simulink model "gnc"  (R2025b)
settings: Solver=ode2  StartTime=0.0  StopTime=inf  FixedStep=1/100  RelTol=1e-3
PreLoadFcn:
  | gnc_PreLoadFcn
undefined symbols (not defined in the file or in its folder): DiscIntNeverNeededParam, dspblkCoreblockFVToolHelper, gcbh
libraries: simulink_extras x7, simulink x5, eeGeneralControl x5
(part 1 of 4)
settings Model: Creator=ac112430  LastModifiedBy=ac124458
settings SolverCC: AlgebraicLoopSolver=TrustRegion
settings DataIOCC: ReturnWorkspaceOutputs=off
settings OptimizationCC: DefaultParameterBehavior=Inlined  DefaultUnderspecifiedDataType=single  PassReuseOutputArgsAs=Individual arguments  DifferentSizesBufferReuse=on  EfficientTunableParamExpr=on
settings DebuggingCC: ParameterPrecisionLossMsg=none  ParameterTunabilityLossMsg=error  UnconnectedInputMsg=warning  UnconnectedOutputMsg=warning  UnconnectedLineMsg=warning  BusObjectLabelMismatch=none  ArithmeticOperatorsInVariantConditions=warning
settings HardwareCC: ProdBitPerPointer=32.0  ProdBitPerSizeT=32.0  ProdBitPerPtrDiffT=32.0  ProdLargestAtomicInteger=Long  ProdLargestAtomicFloat=Double  ProdIntDivRoundTo=Undefined  ProdWordSize=32.0  ProdLongLongMode=on  ProdHWDeviceType=ARM Compatible->ARM Cortex
settings ModelReferenceCC: EnableRefExpFcnMdlSchedulingChecks=on  ModelReferenceNumInstancesAllowed=Single  PropagateSignalLabelsOutOfModel=off
settings SFSimCC: SimUseLocalCustomCode=off  MATLABDynamicMemAlloc=off  CustomCodeUndefinedFunction=UseInterfaceOnly
settings RTWCC: SystemTargetFile=ert.tlc  GenCodeOnly=on  TemplateMakefile=ert_default_tmf  RTWUseLocalCustomCode=off  IncludeHyperlinkInReport=on  GPUComputeCapability=3.5  Description=Embedded Coder
settings CodeAppCC: IgnoreCustomStorageClasses=off  MaxIdLength=2048.0  StateflowObjectComments=on
settings ERTTargetCC: ERTCustomFileTemplate=example_file_process.tlc  ConvertIfToSwitch=off  SuppressUnreachableDefaultCases=off  DynamicArrayContainerType=coder::array  TargetLangStandard=C99 (ISO)  GenerateSampleERTMain=on  SupportComplex=off  SupportVariableSizeSignals=on

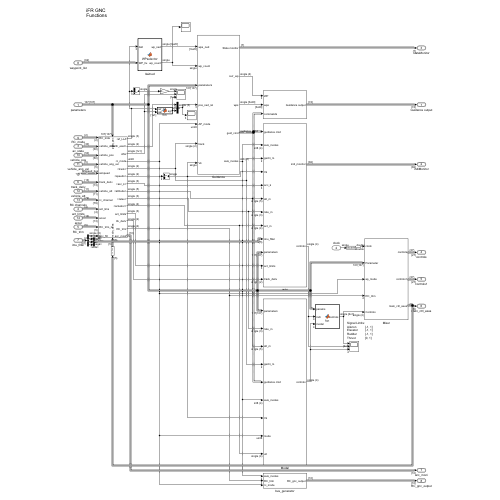
[thumbnail: Simulink's stored preview of the top-level diagram]
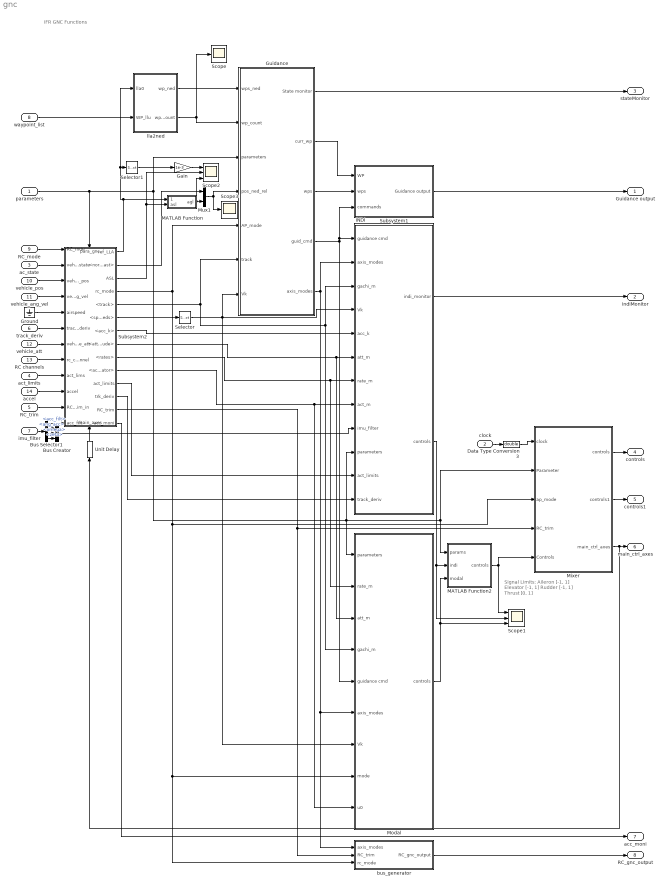
== system gnc ==
  note: iFR GNC Functions
  note: Signal Limits:
      | Aileron		[-1, 1]
      | Elevator		[-1, 1]
      | Rudder		[-1, 1]
      | Thrust		[0, 1]
  parameters : Inport  OutDataTypeStr=Bus: gnc_parameterBus
  clock : Inport  Port=2  OutDataTypeStr=single
  ac_state : Inport  Port=3  OutDataTypeStr=Bus: vehicle_state_bus  PortDimensions=1  SampleTime=[0.01,0]
  act_limits : Inport  Port=4  OutDataTypeStr=Bus: actuator_limits_bus
  RC_trim : Inport  Port=5  OutDataTypeStr=Bus: rc_trim_bus
  track_deriv : Inport  Port=6  OutDataTypeStr=Bus: track_deriv_monitor_bus
  imu_filter : Inport  Port=7  OutDataTypeStr=Bus: ifr_imu_filtered_bus
  waypoint_list : Inport  Port=8  OutDataTypeStr=Bus: waypoint_list_bus
  RC_mode : Inport  Port=9  OutDataTypeStr=Bus: rc_mode_bus
  vehicle_pos : Inport  Port=10  OutDataTypeStr=Bus: vehicle_local_position_bus
  vehicle_ang_vel : Inport  Port=11  OutDataTypeStr=Bus: vehicle_angular_velocity_bus
  vehicle_att : Inport  Port=12  OutDataTypeStr=Bus: vehicle_attitude_bus
  RC channels : Inport  Port=13  OutDataTypeStr=Bus: rc_channels_bus
  accel : Inport  Port=14  OutDataTypeStr=Bus: sensor_accel_bus
  Bus Creator : BusCreator  Inputs=3
  Bus Selector1 : BusSelector  OutputSignals=acc_filt,ang_acc,omega,zeta
  Data Type Conversion3 : DataTypeConversion  OutDataTypeStr=double  SaturateOnIntegerOverflow=off  RndMeth=Floor
  Gain : Gain  Gain=1e-3
  Ground : Ground
  Guidance : Subsystem
  INDI : Subsystem
  MATLAB Function : MATLAB Function  TreatAsAtomicUnit=on
  MATLAB Function2 : MATLAB Function  TreatAsAtomicUnit=on
  Mixer : Subsystem
  Modal : Subsystem
  Mux1 : Mux  Inputs=2
  Scope : Scope
      settings: ActiveDisplayYMinimum=3  ActiveDisplayYMaximum=5  DataLoggingVariableName=ScopeData30
  Scope1 : Scope  NumInputPorts=3
      settings: ActiveDisplayYMinimum=-1  ActiveDisplayYMaximum=1  DataLoggingVariableName=ScopeData2
  Scope2 : Scope  NumInputPorts=3
      settings: ActiveDisplayYMinimum=-356.19794621595673  ActiveDisplayYMaximum=-350.06711072766188  DataLoggingVariableName=ScopeData4
  Scope3 : Scope
      settings: ActiveDisplayYMinimum=-769.31696  ActiveDisplayYMaximum=477.87848  DataLoggingVariableName=ScopeData5
  Selector : Selector  InputPortWidth=2  IndexOptions=Index vector (dialog)  Indices=1  OutputSizes=1
  Selector1 : Selector  InputPortWidth=3  IndexOptions=Index vector (dialog)  Indices=3  OutputSizes=1
  Subsystem1 : Subsystem
  Subsystem2 : Subsystem
      settings: PortSchema="{\"entries\":[{\"content\":{\"sides\":[{\"content\":{\"connectorIds\":[\"In1\",\"In2\",\"In3\",\"In4\",\"In5\",\"In6\",\"In7\",\"In8\",\"In9\",\"In10\",\"In11\",\"In12\"]},\"type\":\"ConnectorPlacement.EquallySpacedRectSide\",\"uuid\":\"eae11f8f-df23-443f-af8c-32e17e4605f0\"},{\"content\":{\"connectorIds\":[\"Out1\",\"Out2\",\"Out3\",\"Out4\",\"Out5\",\"Out6\",\"Out7\",\"Out8\",\"Out9\",\"Out10\",\"Out11\",\"Out12\",\"Out13\",\"Out14\"],\"side\":\"RIGHT\"},\"type\":\"ConnectorPlacement.EquallySpacedRectSide\",\"uuid\":\"25c6a971-14b0-4ed1-9e4e-a0a3a34e6a3d\"},{\"content\":{\"connectorIds\":[\"In13\"],\"side\":\"TOP\"},\"type\":\"ConnectorPlacement.EquallySpacedRectSide\",\"uuid\":\"38764348-8a10-4184-b281-810ae850f533\"},{\"content\":{\"connectorIds\":[\"In14\"],\"side\":\"BOTTOM\"},\"type\":\"ConnectorPlacement.EquallySpacedRectSide\",\"uuid\":\"a4d29612-f53e-4299-8f37-c5a613e7ffff\"}]},\"type\":\"ConnectorPlacement.EquallySpacedConnector\",\"uuid\":\"9dbe3133-1740-4116-b0d1-43b1503b7370\"}],\"packageUris\":[\"http://schema.mathworks.com/mf0/Connector/R2020b\"],\"version\":\"1.0\"}"
  Unit Delay : UnitDelay  SampleTime=-1  HasFrameUpgradeWarning=on
  bus_generator : Subsystem
  lla2ned : MATLAB Function  TreatAsAtomicUnit=on
  Guidance output : Outport  OutDataTypeStr=Bus: guidance_output_bus
  indiMonitor : Outport  Port=2  OutDataTypeStr=Bus: indi_monitor_bus
  stateMonitor : Outport  Port=3  OutDataTypeStr=Bus: guidance_state_bus
  controls : Outport  Port=4  OutDataTypeStr=Bus: actuator_controls_0_bus  VectorParamsAs1DForOutWhenUnconnected=off
  controls1 : Outport  Port=5  OutDataTypeStr=Bus: actuator_controls_1_bus  VectorParamsAs1DForOutWhenUnconnected=off
  main_ctrl_axes : Outport  Port=6  OutDataTypeStr=Bus: main_ctrl_axes_bus
  acc_moni : Outport  Port=7  OutDataTypeStr=Bus: accel_monitor_bus
  RC_gnc_output : Outport  Port=8  OutDataTypeStr=Bus: rc_gnc_output_bus
  wires:
  clock/1 -> Data Type Conversion3/1
  INDI/2(controls) -> Scope1/2, MATLAB Function2/2(indi)
  Subsystem1/1(Guidance output) -> Guidance output/1
  Mixer/1(controls) -> controls/1
  Guidance/1(State monitor) -> stateMonitor/1
  INDI/1(indi_monitor) -> indiMonitor/1
  Data Type Conversion3/1 -> Mixer/1(clock)
  waypoint_list/1 -> lla2ned/2(WP_llu)
  Guidance/4(guid_cmd) -> INDI/1(guidance cmd), Subsystem1/3(commands), Modal/5(guidance cmd)
  Guidance/2(curr_wp) -> Subsystem1/1(WP)
  lla2ned/1(wp_ned) -> Guidance/1(wps_ned)
  Mux1/1 -> Scope3/1, Guidance/4(pos_ned_rel)
  MATLAB Function/1(agl) -> Scope2/3, Mux1/2
  Subsystem2/6(<speeds>) -> Selector/1
  Selector/1 -> Modal/7(Vk), INDI/4(Vk), Guidance/7(Vk)
  lla2ned/2(wp_count) -> Scope/1, Guidance/2(wp_count)
  Subsystem2/11(act_limits) -> INDI/11(act_limits)
  Subsystem2/13(RC_trim) -> Mixer/4(RC_trim), bus_generator/2(RC_trim)
  Mixer/2(controls1) -> controls1/1
  Subsystem2/7(<acc_k>) -> INDI/5(acc_k)
  Subsystem2/8(<attitude>) -> Modal/3(att_m), INDI/6(att_m)
  Subsystem2/5(<track>) -> Modal/4(gachi_m), INDI/3(gachi_m), Guidance/6(track)
  Subsystem2/2(<north_east>) -> Mux1/1
  Subsystem2/9(<rates>) -> Modal/2(rate_m), INDI/7(rate_m)
  Subsystem2/10(<actuator>) -> Modal/9(u0), INDI/8(act_m)
  Guidance/3(wps) -> Subsystem1/2(wps)
  parameters/1 -> Subsystem2/13(para_gnc), Guidance/3(parameters), INDI/10(parameters), Modal/1(parameters), Mixer/2(Parameter), MATLAB Function2/1(params)
  Subsystem2/12(trk_deriv) -> INDI/12(track_deriv)
  Bus Creator/1 -> INDI/9(imu_filter)
  Modal/1(controls) -> Scope1/3, MATLAB Function2/3(modal)
  MATLAB Function2/1(controls) -> Mixer/5(Controls), Scope1/1
  Subsystem2/1(ref_LLA) -> Selector1/1, lla2ned/1(lla0), MATLAB Function/1(ref_lla)
  Subsystem2/3(ASL) -> Scope2/2, MATLAB Function/2(asl)
  Guidance/5(axis_modes) -> bus_generator/1(axis_modes), Modal/6(axis_modes), INDI/2(axis_modes)
  Gain/1 -> Scope2/1
  Selector1/1 -> Gain/1
  Mixer/3(main_ctrl_axes) -> Unit Delay/1, main_ctrl_axes/1
  vehicle_ang_vel/1 -> Subsystem2/4(vehicle_ang_vel)
  Bus Selector1/1 -> Subsystem2/12(acc_filt)  "<acc_filt>"
  RC_mode/1 -> Subsystem2/1(RC_mde)
  act_limits/1 -> Subsystem2/9(act_lims)
  accel/1 -> Subsystem2/10(accel)
  vehicle_pos/1 -> Subsystem2/3(vehicle_pos)
  Unit Delay/1 -> Subsystem2/14(main_axes)
  track_deriv/1 -> Subsystem2/6(track_deriv)
  RC channels/1 -> Subsystem2/8(rc_channel)
  Bus Selector1/4 -> Bus Creator/3  "<zeta>"
  imu_filter/1 -> Bus Selector1/1
  Bus Selector1/3 -> Bus Creator/2  "<omega>"
  vehicle_att/1 -> Subsystem2/7(vehicle_att)
  ac_state/1 -> Subsystem2/2(vehicle_state)
  Bus Selector1/2 -> Bus Creator/1  "<ang_acc>"
  RC_trim/1 -> Subsystem2/11(RC_trim_in)
  Ground/1 -> Subsystem2/5(airspeed)
  Subsystem2/14(acc_moni) -> acc_moni/1
  bus_generator/1(RC_gnc_output) -> RC_gnc_output/1
  Subsystem2/4(rc_mode) -> Guidance/5(AP_mode), bus_generator/3(rc_mode), Modal/8(mode), Mixer/3(ap_mode)

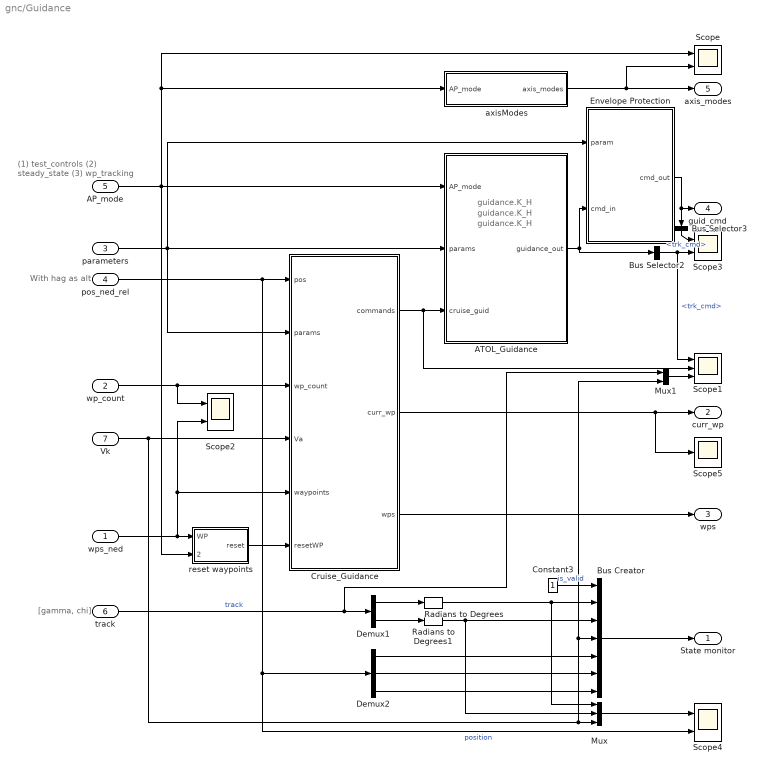
== system gnc/Guidance ==
  note: (1) test_controls
      | (2) steady_state
      | (3) wp_tracking
  note: guidance.K_H
  note: guidance.K_H
  note: guidance.K_H
  note: guidance.K_H
  note: guidance.K_H
  note: With hag as alt
  note: [gamma, chi]
  wps_ned : Inport  PortDimensions=[3,20]
  wp_count : Inport  Port=2  OutDataTypeStr=single
  parameters : Inport  Port=3  OutDataTypeStr=Bus: gnc_parameterBus
  pos_ned_rel : Inport  Port=4
  AP_mode : Inport  Port=5  OutDataTypeStr=uint8  PortDimensions=1
  track : Inport  Port=6  OutDataTypeStr=single  PortDimensions=2
  Vk : Inport  Port=7  OutDataTypeStr=single  PortDimensions=1
  ATOL_Guidance : MATLAB Function  TreatAsAtomicUnit=on
  Bus Creator : BusCreator  Inputs=7
  Bus Selector2 : BusSelector  OutputSignals=trk_cmd
  Bus Selector3 : BusSelector  OutputSignals=trk_cmd
  Constant3 : Constant  OutDataTypeStr=boolean
  Cruise_Guidance : MATLAB Function  TreatAsAtomicUnit=on
  Demux1 : Demux  Outputs=2
  Demux2 : Demux  Outputs=3
  Envelope Protection : MATLAB Function  TreatAsAtomicUnit=on
  Mux : Mux  Inputs=3
  Mux1 : Mux  Inputs=2
  Radians to Degrees : simulink_extras/Transformations/Radians to Degrees
  Radians to Degrees1 : simulink_extras/Transformations/Radians to Degrees
  Scope{,2..4} (4 alike) : Scope  NumInputPorts=2
      Scope settings: ActiveDisplayYMinimum=-0.70542635658915032  ActiveDisplayYMaximum=4.5271317829457374  DataLoggingVariableName=ScopeData7
      Scope2 settings: ActiveDisplayYMinimum=-139.15896797180176  ActiveDisplayYMaximum=109.10070991516113  DataLoggingVariableName=ScopeData29
      Scope3 settings: ActiveDisplayYMinimum=-1.4161849710982644  ActiveDisplayYMaximum=1.5643063583815042  DataLoggingVariableName=ScopeData2
      Scope4 settings: ActiveDisplayYMinimum=-139.15896797180176  ActiveDisplayYMaximum=109.10070991516113  DataLoggingVariableName=ScopeData3
  Scope1 : Scope  NumInputPorts=3
      settings: ActiveDisplayYMinimum=-2.4999999999999996  ActiveDisplayYMaximum=22.5  DataLoggingVariableName=ScopeData12
  Scope5 : Scope
      settings: ActiveDisplayYMinimum=-6.4510081708431244  ActiveDisplayYMaximum=26.644176095724106  DataLoggingVariableName=ScopeData31
  axisModes : MATLAB Function  TreatAsAtomicUnit=on
  reset waypoints : MATLAB Function  TreatAsAtomicUnit=on
  State monitor : Outport  OutDataTypeStr=Bus: guidance_state_bus
  curr_wp : Outport  Port=2  PortDimensions=4
  wps : Outport  Port=3  OutDataTypeStr=single  PortDimensions=[3,20]
  guid_cmd : Outport  Port=4  OutDataTypeStr=Bus: guidance_cmd
  axis_modes : Outport  Port=5  OutDataTypeStr=int8  PortDimensions=4  LockScale=on
  wires:
  Constant3/1 -> Bus Creator/1  "is_valid"
  Vk/1 -> Mux1/2, Bus Creator/4, Mux/3, Cruise_Guidance/4(Va)
  Mux/1 -> Scope4/1
  Demux2/2 -> Bus Creator/6
  Demux2/1 -> Bus Creator/5
  Demux2/3 -> Bus Creator/7
  wps_ned/1 -> Scope2/2, Cruise_Guidance/5(waypoints), reset waypoints/1(WP)
  Demux1/1 -> Radians to Degrees/1
  track/1 -> Mux1/1, Demux1/1  "track"
  Demux1/2 -> Radians to Degrees1/1
  Cruise_Guidance/2(curr_wp) -> Scope5/1, curr_wp/1
  Bus Creator/1 -> State monitor/1
  reset waypoints/1(reset) -> Cruise_Guidance/6(resetWP)
  pos_ned_rel/1 -> Demux2/1, Scope4/2, Cruise_Guidance/1(pos)  "position"
  ATOL_Guidance/1(guidance_out) -> Envelope Protection/2(cmd_in), Bus Selector2/1
  Radians to Degrees/1 -> Bus Creator/2, Mux/1
  Radians to Degrees1/1 -> Mux/2, Bus Creator/3
  parameters/1 -> Envelope Protection/1(param), ATOL_Guidance/2(params), Cruise_Guidance/2(params)
  Envelope Protection/1(cmd_out) -> guid_cmd/1, Bus Selector3/1
  Cruise_Guidance/1(commands) -> Scope1/2, ATOL_Guidance/3(cruise_guid)
  wp_count/1 -> Scope2/1, Cruise_Guidance/3(wp_count)
  AP_mode/1 -> reset waypoints/2(cruise_sw), Scope/1, axisModes/1(AP_mode), ATOL_Guidance/1(AP_mode)
  Bus Selector2/1 -> Scope1/1, Scope3/2  "<trk_cmd>"
  Bus Selector3/1 -> Scope3/1  "<trk_cmd>"
  Cruise_Guidance/3(wps) -> wps/1
  axisModes/1(axis_modes) -> Scope/2, axis_modes/1
  Mux1/1 -> Scope1/3

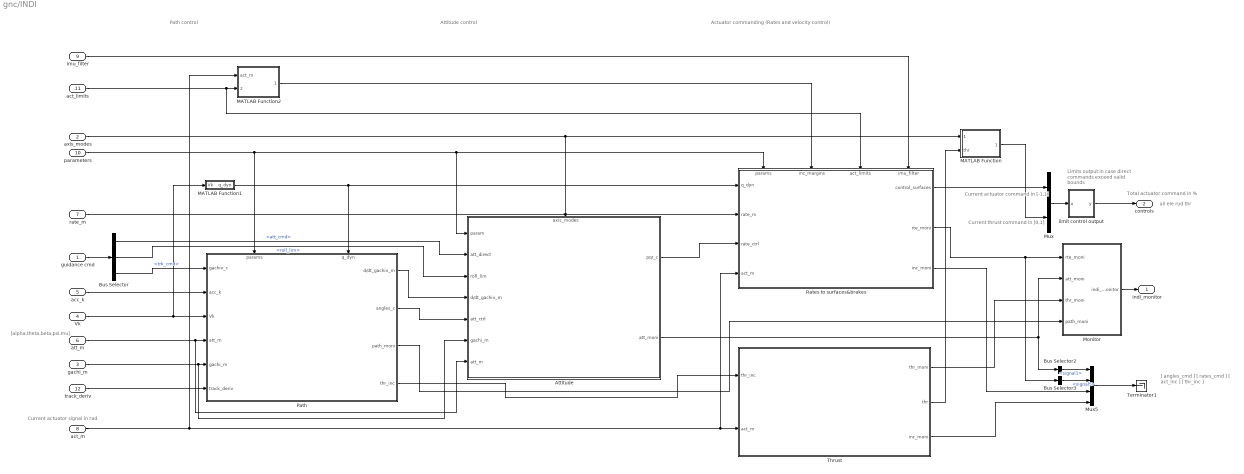
== system gnc/INDI ==
  note: [ angles_cmd	]
      | [ rates_cmd	]
      | [ act_inc		]
      | [ thr_inc		]
  note: ail ele rud thr
  note: Path control
  note: Current actuator
      | signal in rad
  note: [alpha,theta,beta,psi,mu]
  note: Attitude control
  note: Actuator commanding (Rates and velocity control)
  note: Limits output in case
      | direct commands
      | exceed valid bounds
  note: Current thrust command in [0,1]
  note: Total actuator
      | command in %
  note: Current actuator command in [-1,1]
  guidance cmd : Inport  OutDataTypeStr=Bus: guidance_cmd
  axis_modes : Inport  Port=2  OutDataTypeStr=int8
  gachi_m : Inport  Port=3
  Vk : Inport  Port=4  PortDimensions=1
  acc_k : Inport  Port=5
  att_m : Inport  Port=6  OutDataTypeStr=single  PortDimensions=5
  rate_m : Inport  Port=7  OutDataTypeStr=single  PortDimensions=3
  act_m : Inport  Port=8  OutDataTypeStr=single  PortDimensions=4
  imu_filter : Inport  Port=9
  parameters : Inport  Port=10  OutDataTypeStr=Bus: gnc_parameterBus
  act_limits : Inport  Port=11
  track_deriv : Inport  Port=12  OutDataTypeStr=single  PortDimensions=2
  Attitude : Subsystem
      settings: PortSchema="{\"entries\":[{\"content\":{\"sides\":[{\"content\":{\"connectorIds\":[\"In1\",\"In2\",\"In3\",\"In4\",\"In5\",\"In6\",\"In7\"]},\"type\":\"ConnectorPlacement.EquallySpacedRectSide\",\"uuid\":\"b7c7e1a9-3024-403b-8101-4fc7eff0575e\"},{\"content\":{\"connectorIds\":[\"Out1\",\"Out2\"],\"side\":\"RIGHT\"},\"type\":\"ConnectorPlacement.EquallySpacedRectSide\",\"uuid\":\"cb53e122-7831-4c34-8aea-2b31ecc7af3b\"},{\"content\":{\"connectorIds\":[\"In8\"],\"side\":\"TOP\"},\"type\":\"ConnectorPlacement.EquallySpacedRectSide\",\"uuid\":\"4b53ef0a-efac-44dd-914a-4d2217d9826d\"}]},\"type\":\"ConnectorPlacement.EquallySpacedConnector\",\"uuid\":\"b88ec9b5-5f11-4970-871c-b4ff42b920b3\"}],\"packageUris\":[\"http://schema.mathworks.com/mf0/Connector/R2020b\"],\"version\":\"1.0\"}"
  Bus Selector : BusSelector  OutputSignals=att_cmd,roll_lim,trk_cmd
  Bus Selector2 : BusSelector  OutputSignals=signal1
  Bus Selector3 : BusSelector  OutputSignals=signal1.signal5
  MATLAB Function : MATLAB Function  TreatAsAtomicUnit=on
  MATLAB Function1 : MATLAB Function  TreatAsAtomicUnit=on
  MATLAB Function2 : MATLAB Function  TreatAsAtomicUnit=on
  Monitor : Subsystem
  Mux : Mux  Inputs=2
  Mux5 : Mux
  Path : Subsystem
      settings: PortSchema="{\"entries\":[{\"content\":{\"sides\":[{\"content\":{\"connectorIds\":[\"In1\",\"In2\",\"In3\",\"In4\",\"In5\",\"In6\"]},\"type\":\"ConnectorPlacement.EquallySpacedRectSide\",\"uuid\":\"aeeb4c65-4157-49e3-89f2-8442de4c35c3\"},{\"content\":{\"connectorIds\":[\"Out1\",\"Out2\",\"Out3\",\"Out4\"],\"side\":\"RIGHT\"},\"type\":\"ConnectorPlacement.EquallySpacedRectSide\",\"uuid\":\"9484377b-093c-4072-8beb-471d4a7ab8a9\"},{\"content\":{\"connectorIds\":[\"In7\",\"In8\"],\"side\":\"TOP\"},\"type\":\"ConnectorPlacement.EquallySpacedRectSide\",\"uuid\":\"c6253d73-40c9-4522-8e2e-6cc388a7bc53\"},{\"content\":{\"side\":\"BOTTOM\"},\"type\":\"ConnectorPlacement.EquallySpacedRectSide\",\"uuid\":\"b5f53673-25a9-4222-bcda-17be59006191\"}]},\"type\":\"ConnectorPlacement.EquallySpacedConnector\",\"uuid\":\"6ddcfaaa-ad15-4bea-bdab-3495e7fd8cf9\"}],\"packageUris\":[\"http://schema.mathworks.com/mf0/Connector/R2020b\"],\"version\":\"1.0\"}"
  Rates to surfaces&brakes : Subsystem
      settings: PortSchema="{\"entries\":[{\"content\":{\"sides\":[{\"content\":{\"connectorIds\":[\"In1\",\"In2\",\"In3\",\"In4\"]},\"type\":\"ConnectorPlacement.EquallySpacedRectSide\",\"uuid\":\"38e84281-7140-4c55-a86a-c71fe3b9f0d7\"},{\"content\":{\"connectorIds\":[\"Out1\",\"Out2\",\"Out3\"],\"side\":\"RIGHT\"},\"type\":\"ConnectorPlacement.EquallySpacedRectSide\",\"uuid\":\"18979a8d-3905-4a49-86c3-949277d06de1\"},{\"content\":{\"connectorIds\":[\"In5\",\"In6\",\"In7\",\"In8\"],\"side\":\"TOP\"},\"type\":\"ConnectorPlacement.EquallySpacedRectSide\",\"uuid\":\"2ae550e8-8587-46c8-a90f-db3ecfdcb8e8\"},{\"content\":{\"side\":\"BOTTOM\"},\"type\":\"ConnectorPlacement.EquallySpacedRectSide\",\"uuid\":\"d561a624-fdf7-40a1-bac0-8ec2b91f5f36\"}]},\"type\":\"ConnectorPlacement.EquallySpacedConnector\",\"uuid\":\"df4b2bf7-ea7e-4f09-bf8e-e1a831543136\"}],\"packageUris\":[\"http://schema.mathworks.com/mf0/Connector/R2020b\"],\"version\":\"1.0\"}"
  Terminator1 : Terminator
  Thrust : Subsystem
  limit control output : MATLAB Function  TreatAsAtomicUnit=on
  indi_monitor : Outport  OutDataTypeStr=Bus: indi_monitor_bus
  controls : Outport  Port=2  OutDataTypeStr=single  PortDimensions=4  VectorParamsAs1DForOutWhenUnconnected=off
  wires:
  Bus Selector/2 -> Attitude/3(roll_lim)  "<roll_lim>"
  Thrust/3(inc_moni) -> Mux5/4
  Path/3(path_moni) -> Monitor/4(path_moni)
  Rates to surfaces&brakes/3(inc_moni) -> Mux5/3
  parameters/1 -> Rates to surfaces&brakes/5(params), Attitude/1(param), Path/7(params)
  Mux5/1 -> Terminator1/1
  att_m/1 -> Attitude/7(att_m), Path/4(att_m)
  acc_k/1 -> Path/2(acc_k)
  Rates to surfaces&brakes/1(control_surfaces) -> Mux/1
  Bus Selector/3 -> Path/1(gachiv_c)  "<trk_cmd>"
  Attitude/1(pqr_c) -> Rates to surfaces&brakes/3(rate_ctrl)
  Vk/1 -> MATLAB Function1/1(Vk), Path/3(Vk)
  act_m/1 -> Thrust/2(act_m), Rates to surfaces&brakes/4(act_m), MATLAB Function2/1(act_m)
  Path/4(thr_inc) -> Thrust/1(thr_inc)
  rate_m/1 -> Rates to surfaces&brakes/2(rate_m)
  Path/2(angles_c) -> Attitude/5(att_ctrl)
  Thrust/2(thr) -> MATLAB Function/2(thr)
  guidance cmd/1 -> Bus Selector/1
  Path/1(d/dt_gachiv_m) -> Attitude/4(d/dt_gachiv_m)
  Thrust/1(thr_moni) -> Monitor/3(thr_moni)
  Rates to surfaces&brakes/2(rte_moni) -> Monitor/1(rte_moni), Bus Selector3/1
  gachi_m/1 -> Attitude/6(gachi_m), Path/5(gachi_m)
  Monitor/1(indi_monitor) -> indi_monitor/1
  Bus Selector2/1 -> Mux5/1  "<signal1>"
  Bus Selector3/1 -> Mux5/2  "<signal5>"
  Attitude/2(att_moni) -> Monitor/2(att_moni), Bus Selector2/1
  track_deriv/1 -> Path/6(track_deriv)
  limit control output/1(y) -> controls/1
  act_limits/1 -> Rates to surfaces&brakes/7(act_limits), MATLAB Function2/2(act_limit)
  MATLAB Function2/1(inc_margins) -> Rates to surfaces&brakes/6(inc_margins)
  imu_filter/1 -> Rates to surfaces&brakes/8(imu_filter)
  Mux/1 -> limit control output/1(u)
  axis_modes/1 -> MATLAB Function/1(axis_modes), Attitude/8(axis_modes)
  MATLAB Function/1(thr_cmd) -> Mux/2
  Bus Selector/1 -> Attitude/2(att_direct)  "<att_cmd>"
  MATLAB Function1/1(q_dyn) -> Rates to surfaces&brakes/1(q_dyn), Path/8(q_dyn)

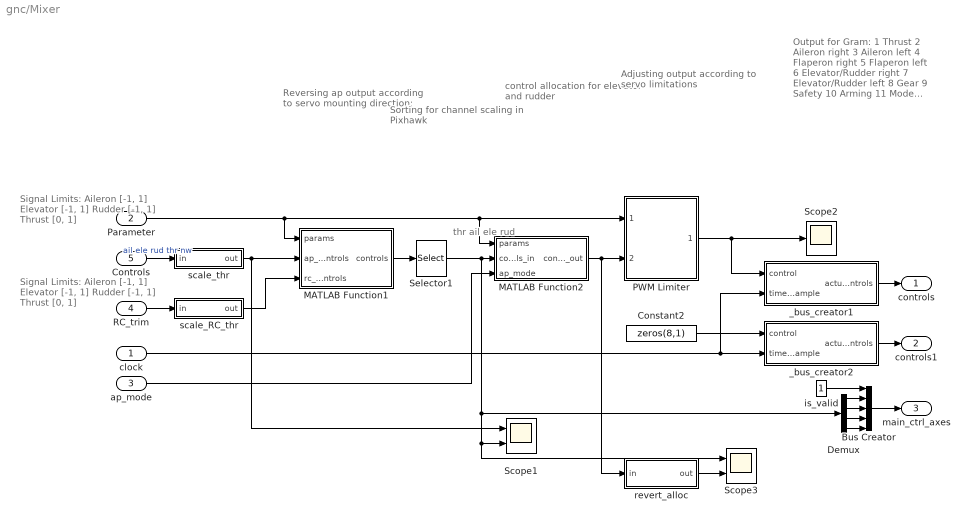
== system gnc/Mixer ==
  note: control allocation for elevator and rudder
  note: Reversing ap output according to servo mounting direction;
  note: Adjusting output
      | according to servo
      | limitations
  note: Sorting for channel
      | scaling in Pixhawk
  note: thr
      | ail
      | ele
      | rud
  note: Output for Gram:
      | 1 Thrust
      | 2 Aileron right
      | 3 Aileron left
      | 4 Flaperon right
      | 5 Flaperon left
      | 6 Elevator/Rudder right
      | 7 Elevator/Rudder left
      | 8 Gear
      | 9 Safety
      | 10 Arming
      | 11 Mode switch
  note: Signal Limits:
      | Aileron		[-1, 1]
      | Elevator		[-1, 1]
      | Rudder		[-1, 1]
      | Thrust		[0, 1]
  note: Signal Limits:
      | Aileron		[-1, 1]
      | Elevator		[-1, 1]
      | Rudder		[-1, 1]
      | Thrust		[0, 1]
  clock : Inport  OutDataTypeStr=double
  Parameter : Inport  Port=2  OutDataTypeStr=Bus: gnc_parameterBus
  ap_mode : Inport  Port=3
  RC_trim : Inport  Port=4
  Controls : Inport  Port=5  OutDataTypeStr=single  PortDimensions=4
  Bus Creator : BusCreator  Inputs=5  OutDataTypeStr=Bus: main_ctrl_axes_bus
      settings: InheritFromInputs=off
  Constant2 : Constant  Value=zeros(8,1)  OutDataTypeStr=single
  Demux : Demux
  MATLAB Function1 : MATLAB Function  TreatAsAtomicUnit=on
  MATLAB Function2 : MATLAB Function  TreatAsAtomicUnit=on
  PWM Limiter : MATLAB Function  TreatAsAtomicUnit=on
  Scope1 : Scope  NumInputPorts=2
      settings: ActiveDisplayYMinimum=-1.25  ActiveDisplayYMaximum=1.25  DataLoggingVariableName=ScopeData8
  Scope2 : Scope
      settings: ActiveDisplayYMinimum=-2.2855338454246521  ActiveDisplayYMaximum=2.2855338454246521  DataLoggingVariableName=ScopeData2
  Scope3 : Scope  NumInputPorts=2
      settings: ActiveDisplayYMinimum=-1.25  ActiveDisplayYMaximum=1.25  DataLoggingVariableName=ScopeData13
  Selector1 : Selector  InputPortWidth=4  IndexOptions=Index vector (dialog)  Indices=[4 1 2 3]  OutputSizes=1
  _bus_creator1 : Subsystem
  _bus_creator2 : Subsystem
  is_valid : Constant  OutDataTypeStr=boolean
  revert_alloc : MATLAB Function  TreatAsAtomicUnit=on
  scale_RC_thr : MATLAB Function  TreatAsAtomicUnit=on
  scale_thr : MATLAB Function  TreatAsAtomicUnit=on
  controls : Outport  OutDataTypeStr=Bus: actuator_controls_0_bus  VectorParamsAs1DForOutWhenUnconnected=off
  controls1 : Outport  Port=2  OutDataTypeStr=Bus: actuator_controls_bus  VectorParamsAs1DForOutWhenUnconnected=off
  main_ctrl_axes : Outport  Port=3  OutDataTypeStr=Bus: main_ctrl_axes_bus
  wires:
  Controls/1 -> scale_thr/1(in)  "ail ele rud thr nw"
  Parameter/1 -> MATLAB Function2/1(params), PWM Limiter/1(parameter), MATLAB Function1/1(params)
  PWM Limiter/1(controlsLtd) -> _bus_creator1/1(control), Scope2/1
  clock/1 -> _bus_creator2/2(timestamp_sample), _bus_creator1/2(timestamp_sample)
  RC_trim/1 -> scale_RC_thr/1(in)
  _bus_creator1/1(actuator_controls) -> controls/1
  _bus_creator2/1(actuator_controls) -> controls1/1
  Constant2/1 -> _bus_creator2/1(control)
  scale_RC_thr/1(out) -> MATLAB Function1/3(rc_controls)
  MATLAB Function1/1(controls) -> Selector1/1
  scale_thr/1(out) -> MATLAB Function1/2(ap_controls), Scope1/1
  is_valid/1 -> Bus Creator/1
  Demux/1 -> Bus Creator/2
  Demux/2 -> Bus Creator/3
  Demux/3 -> Bus Creator/4
  Demux/4 -> Bus Creator/5
  Bus Creator/1 -> main_ctrl_axes/1
  ap_mode/1 -> MATLAB Function2/3(ap_mode)
  Selector1/1 -> Scope3/1, Scope1/2, Demux/1, MATLAB Function2/2(controls_in)
  MATLAB Function2/1(controls_out) -> revert_alloc/1(in), PWM Limiter/2(controls)
  revert_alloc/1(out) -> Scope3/2

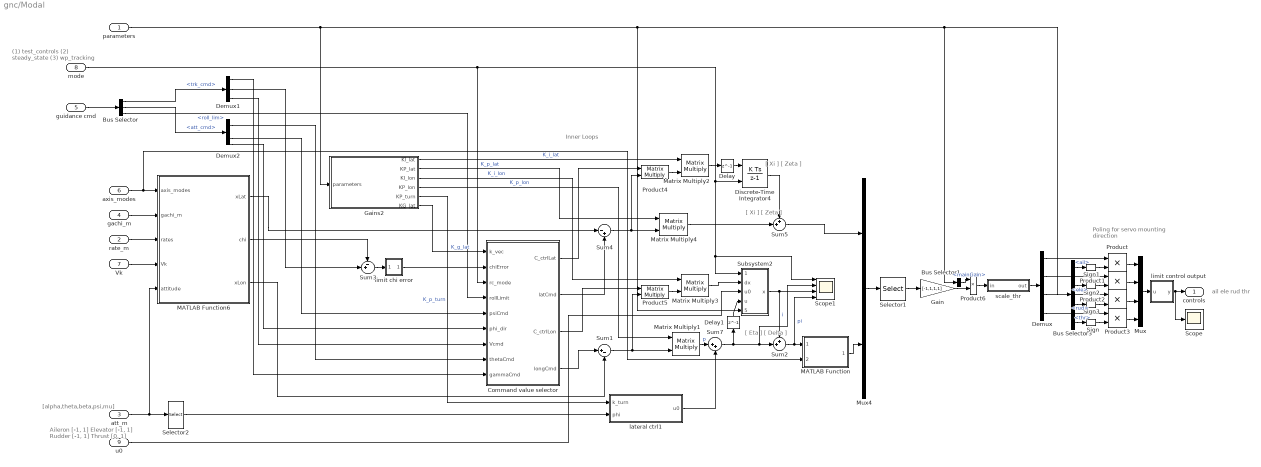
== system gnc/Modal ==
  note: [alpha,theta,beta,psi,mu]
  note: ail ele rud thr
  note: Poling for servo
      | mounting direction
  note: [ Xi     ]
      | [ Zeta ]
  note: Inner Loops
  note: [ Xi     ]
      | [ Zeta ]
  note: [ Eta    ]
      | [ Delta ]
  note: (1) test_controls
      | (2) steady_state
      | (3) wp_tracking
  note: Aileron		[-1, 1]
      | Elevator		[-1, 1]
      | Rudder		[-1, 1]
      | Thrust		[0, 1]
  parameters : Inport  OutDataTypeStr=Bus: gnc_parameterBus
  rate_m : Inport  Port=2  OutDataTypeStr=single  PortDimensions=3
  att_m : Inport  Port=3  OutDataTypeStr=single  PortDimensions=5
  gachi_m : Inport  Port=4
  guidance cmd : Inport  Port=5  OutDataTypeStr=Bus: guidance_cmd
  axis_modes : Inport  Port=6  OutDataTypeStr=int8
  Vk : Inport  Port=7  PortDimensions=1
  mode : Inport  Port=8  OutDataTypeStr=uint8
  u0 : Inport  Port=9  OutDataTypeStr=single  PortDimensions=4
  Bus Selector : BusSelector  OutputSignals=trk_cmd,att_cmd,roll_lim
  Bus Selector1 : BusSelector  OutputSignals=lonCruise.mainGain
  Bus Selector3 : BusSelector  OutputSignals=controlsigns.ail,controlsigns.ele,controlsigns.rud,controlsigns.thr
  Command value selector : MATLAB Function  TreatAsAtomicUnit=on
  Delay : Delay  DelayLength=1
  Delay1 : Delay  DelayLength=1
  Demux : Demux
  Demux1 : Demux  Outputs=3
  Demux2 : Demux  Outputs=5
  Discrete-Time Integrator4 : DiscreteIntegrator  ExternalReset=either  SampleTime=-1  LimitOutput=on  UpperSaturationLimit=15  LowerSaturationLimit=-15  ICPrevOutput=DiscIntNeverNeededParam  ICPrevScaledInput=DiscIntNeverNeededParam
  Gain : Gain  Gain=[-1,1,1,1]
  Gains2 : MATLAB Function  TreatAsAtomicUnit=on
  MATLAB Function : MATLAB Function  TreatAsAtomicUnit=on
  MATLAB Function6 : MATLAB Function  TreatAsAtomicUnit=on
  Matrix Multiply{1..4} (4 alike) : Product  Multiplication=Matrix(*)
  Mux : Mux
  Mux4 : Mux  Inputs=2
  Product{,1..3} (4 alike) : Product  OutDataTypeStr=single
  Product4 : Product  Multiplication=Matrix(*)
  Product5 : Product  Multiplication=Matrix(*)
  Product6 : Product
  Scope : Scope
      settings: DataLoggingVariableName=ScopeData9
  Scope1 : Scope  NumInputPorts=4
      settings: DataLoggingVariableName=ScopeData10
  Selector1 : Selector  InputPortWidth=4  IndexOptions=Index vector (dialog)  Indices=[1,3,2,4]  OutputSizes=1
  Selector2 : Selector  InputPortWidth=5  IndexOptions=Index vector (dialog)  Indices=5  OutputSizes=1
  Sign{,1..3} (4 alike) : Signum
  Subsystem2 : Subsystem
      mask Display:
      | disp('\bf\fontsize{12}\int dx', 'texmode', 'on')
      | port_label('input', 2, 'dx', 'texmode', 'on')
      | port_label('input', 1, 'Tr')
      | port_label('input', 3, 'u_0', 'texmode', 'on')
      | port_label('input', 4, 'u_P', 'texmode', 'on')
      | 
      | port_label('output', 1, 'x', 'texmode', 'on')
  Sum1 : Sum  Inputs=|+-
  Sum2 : Sum  Inputs=++|
  Sum3 : Sum  Inputs=-+|
  Sum4 : Sum  Inputs=|-+
  Sum5 : Sum  Inputs=++|
  Sum7 : Sum  Inputs=|++
  lateral ctrl1 : MATLAB Function  TreatAsAtomicUnit=on
  limit chi error : MATLAB Function  TreatAsAtomicUnit=on
  limit control output : MATLAB Function  TreatAsAtomicUnit=on
  scale_thr : MATLAB Function  TreatAsAtomicUnit=on
  controls : Outport  OutDataTypeStr=single  PortDimensions=4  VectorParamsAs1DForOutWhenUnconnected=off
  wires:
  limit control output/1(y) -> Scope/1, controls/1
  guidance cmd/1 -> Bus Selector/1
  Gain/1 -> Product6/2
  Mux4/1 -> Selector1/1
  Selector1/1 -> Gain/1
  Bus Selector/1 -> Demux1/1  "<trk_cmd>"
  Demux/4 -> Product3/1
  Demux/2 -> Product1/1
  Bus Selector3/3 -> Sign3/1  "<rud>"
  Sign/1 -> Product3/2
  Bus Selector3/1 -> Sign1/1  "<ail>"
  Demux/1 -> Product/1
  Bus Selector3/2 -> Sign2/1  "<ele>"
  Sign1/1 -> Product/2
  Demux/3 -> Product2/1
  Bus Selector3/4 -> Sign/1  "<thr>"
  Sign2/1 -> Product1/2
  Sign3/1 -> Product2/2
  Product/1 -> Mux/1
  Product1/1 -> Mux/2
  Product2/1 -> Mux/3
  Product3/1 -> Mux/4
  Mux/1 -> limit control output/1(u)
  scale_thr/1(out) -> Demux/1
  MATLAB Function/1(ele_thr_cmd) -> Mux4/2
  Bus Selector/2 -> Demux2/1  "<att_cmd>"
  parameters/1 -> Gains2/1(parameters), Bus Selector1/1, Bus Selector3/1, Subsystem2/5(param)
  Sum5/1 -> Mux4/1
  Delay1/1 -> Subsystem2/4(u)
  Delay/1 -> Discrete-Time Integrator4/1
  Command value selector/1(C_ctrlLat) -> Product4/1
  Demux2/4 -> Command value selector/5(psiCmd)
  Gains2/5(KP_turn) -> lateral ctrl1/1(k_turn)  "K_p_turn"
  Product4/1 -> Matrix Multiply2/2
  Gains2/1(KI_lat) -> Matrix Multiply2/1  "K_i_lat"
  Gains2/3(KI_lon) -> Matrix Multiply3/1  "K_i_lon"
  Matrix Multiply1/1 -> Sum7/1  "p"
  Command value selector/2(latCmd) -> Sum4/2
  Gains2/2(KP_lat) -> Matrix Multiply4/1  "K_p_lat"
  Demux1/3 -> Command value selector/7(Vcmd)
  limit chi error/1(y) -> Command value selector/2(chiError)
  Product5/1 -> Matrix Multiply3/2
  Command value selector/4(longCmd) -> Sum1/1
  Demux2/2 -> Command value selector/8(thetaCmd)
  Matrix Multiply3/1 -> Subsystem2/2(dx)
  Command value selector/3(C_ctrlLon) -> Product5/1
  Discrete-Time Integrator4/1 -> Sum5/1
  Demux1/1 -> Command value selector/9(gammaCmd)
  Gains2/4(KP_lon) -> Matrix Multiply1/1  "K_p_lon"
  Subsystem2/1(x) -> Sum2/1, Scope1/3  "i"
  Matrix Multiply2/1 -> Delay/1
  MATLAB Function6/3(xLon) -> Sum1/2
  Sum4/1 -> Product4/2, Matrix Multiply4/2
  lateral ctrl1/1(u0) -> Sum7/2
  MATLAB Function6/1(xLat) -> Sum4/1
  Sum2/1 -> Scope1/4, MATLAB Function/1(ele_thr)  "pi"
  Selector2/1 -> lateral ctrl1/2(phi)
  Bus Selector/3 -> Command value selector/4(rollLimit)  "<roll_lim>"
  u0/1 -> Subsystem2/3(u0)
  Sum3/1 -> limit chi error/1(u)
  Sum1/1 -> Product5/2, Matrix Multiply1/2
  mode/1 -> Discrete-Time Integrator4/2, Scope1/1, Subsystem2/1(mode), Command value selector/3(rc_mode)
  Sum7/1 -> Delay1/1, Scope1/2, Sum2/2
  Matrix Multiply4/1 -> Sum5/2
  MATLAB Function6/2(chi) -> Sum3/1
  att_m/1 -> MATLAB Function6/5(attitude), Selector2/1
  Vk/1 -> MATLAB Function6/4(Vk)
  gachi_m/1 -> MATLAB Function6/2(gachi_m)
  rate_m/1 -> MATLAB Function6/3(rates)
  Demux1/2 -> Sum3/2
  Demux2/5 -> Command value selector/6(phi_dir)
  Gains2/6(KG_lat) -> Command value selector/1(k_vec)  "K_g_lat"
  axis_modes/1 -> MATLAB Function/2(axis_modes), MATLAB Function6/1(axis_modes)
  Product6/1 -> scale_thr/1(in)
  Bus Selector1/1 -> Product6/1  "<mainGain>"

== system gnc/Subsystem1 ==
  note: vCmd
      |
      | chiCmd
      |
      | psiCmd
      |
      | rollLim
      |
      | gammaCmd
      |
      | alphaCmd
  WP : Inport  PortDimensions=4
  wps : Inport  Port=2
  commands : Inport  Port=3  OutDataTypeStr=Bus: guidance_cmd
  Bus Creator2 : BusCreator  Inputs=11  OutDataTypeStr=Bus: guidance_output_bus
  Bus Selector : BusSelector  OutputSignals=trk_cmd,roll_lim,att_cmd
  Constant : Constant  Value=zeros(3,1)  OutDataTypeStr=single
  Demux1 : Demux
  Demux2 : Demux  Outputs=3
  Demux3 : Demux  Outputs=2
  MATLAB Function : MATLAB Function  TreatAsAtomicUnit=on
  Mux : Mux  Inputs=3
  Radians to Degrees{,1..4} (5 alike) : simulink_extras/Transformations/Radians to Degrees
  Selector1 : Selector  InputPortWidth=5  IndexOptions=Index vector (dialog)  Indices=[4 1]  OutputSizes=1
  is_valid : Constant  Value=true  OutDataTypeStr=boolean
  Guidance output : Outport  OutDataTypeStr=Bus: guidance_output_bus
  wires:
  Bus Creator2/1 -> Guidance output/1
  Constant/1 -> Bus Creator2/5  "offset_lat"
  is_valid/1 -> Bus Creator2/1
  Mux/1 -> Bus Creator2/4  "first_wp"
  commands/1 -> Bus Selector/1
  Demux1/1 -> Bus Creator2/3
  WP/1 -> Demux1/1
  Demux1/2 -> Mux/1
  Demux1/3 -> Mux/2
  Demux1/4 -> Mux/3
  Bus Selector/1 -> Demux2/1  "<trk_cmd>"
  Bus Selector/3 -> Selector1/1  "<att_cmd>"
  Demux2/1 -> Radians to Degrees1/1
  Demux2/2 -> Radians to Degrees4/1
  Demux2/3 -> Bus Creator2/6
  Selector1/1 -> Demux3/1
  Demux3/1 -> Radians to Degrees3/1
  Demux3/2 -> Radians to Degrees/1
  Bus Selector/2 -> Radians to Degrees2/1  "<roll_lim>"
  Radians to Degrees/1 -> Bus Creator2/11
  Radians to Degrees1/1 -> Bus Creator2/10
  Radians to Degrees2/1 -> Bus Creator2/9
  Radians to Degrees3/1 -> Bus Creator2/8
  Radians to Degrees4/1 -> Bus Creator2/7
  wps/1 -> MATLAB Function/1(array_in)  "cruise_wps"
  MATLAB Function/1(array_out) -> Bus Creator2/2

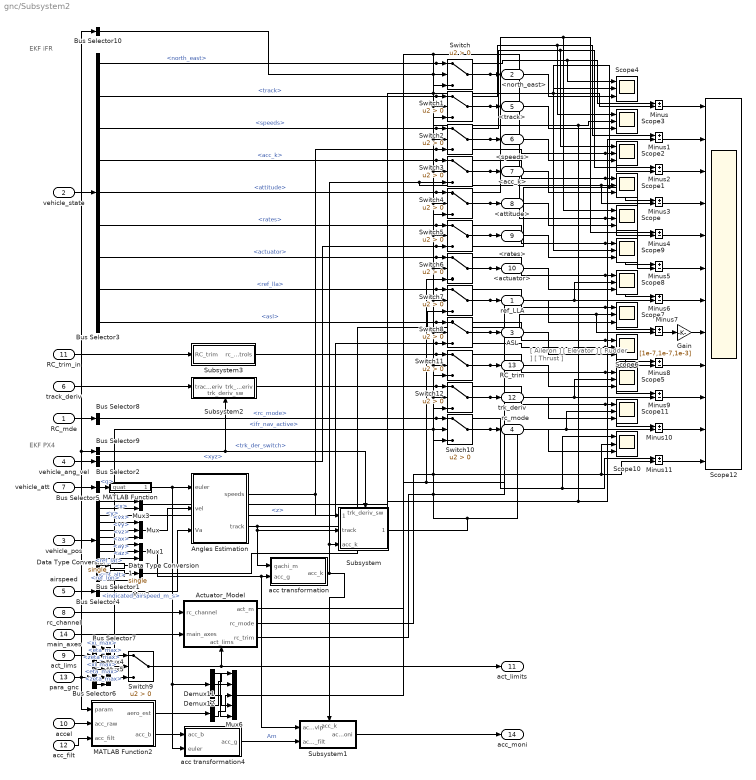
== system gnc/Subsystem2 ==
  note: [ Aileron	  ]
      | [ Elevator ]
      | [ Rudder	  ]
      | [ Thrust	  ]
  note: EKF PX4
  note: EKF iFR
  RC_mde : Inport  OutDataTypeStr=Bus: rc_mode_bus
  vehicle_state : Inport  Port=2  OutDataTypeStr=Bus: vehicle_state_bus
  vehicle_pos : Inport  Port=3  OutDataTypeStr=Bus: vehicle_local_position_bus
  vehicle_ang_vel : Inport  Port=4  OutDataTypeStr=Bus: vehicle_angular_velocity_bus
  airspeed : Inport  Port=5  OutDataTypeStr=Bus: airspeed_bus
  track_deriv : Inport  Port=6  OutDataTypeStr=Bus: track_deriv_monitor_bus
  vehicle_att : Inport  Port=7  OutDataTypeStr=Bus: vehicle_attitude_bus
  rc_channel : Inport  Port=8  OutDataTypeStr=Bus: rc_channels_bus
  act_lims : Inport  Port=9  OutDataTypeStr=Bus: actuator_limits_bus
  accel : Inport  Port=10  OutDataTypeStr=Bus: sensor_accel_bus
  RC_trim_in : Inport  Port=11  OutDataTypeStr=Bus: rc_trim_bus
  acc_filt : Inport  Port=12
  para_gnc : Inport  Port=13  OutDataTypeStr=Bus: gnc_parameterBus
  main_axes : Inport  Port=14  OutDataTypeStr=Bus: main_ctrl_axes_bus
  Actuator_Model : Subsystem
      settings: PortSchema="{\"entries\":[{\"content\":{\"sides\":[{\"content\":{\"connectorIds\":[\"In1\",\"In2\"]},\"type\":\"ConnectorPlacement.EquallySpacedRectSide\",\"uuid\":\"0b560cb0-425b-4e75-ad69-9f3dd2ae247d\"},{\"content\":{\"connectorIds\":[\"Out1\",\"Out2\",\"Out3\"],\"side\":\"RIGHT\"},\"type\":\"ConnectorPlacement.EquallySpacedRectSide\",\"uuid\":\"67043da2-be34-4466-be37-15cebe548400\"},{\"content\":{\"side\":\"TOP\"},\"type\":\"ConnectorPlacement.EquallySpacedRectSide\",\"uuid\":\"dbc9e13d-738a-4a6f-867f-431ba88297cf\"},{\"content\":{\"connectorIds\":[\"In3\"],\"side\":\"BOTTOM\"},\"type\":\"ConnectorPlacement.EquallySpacedRectSide\",\"uuid\":\"14b82ace-20eb-4480-853b-ffa5dbbc5ee0\"}]},\"type\":\"ConnectorPlacement.EquallySpacedConnector\",\"uuid\":\"43045ae4-5565-43c8-8df8-998e069be6cd\"}],\"packageUris\":[\"http://schema.mathworks.com/mf0/Connector/R2020b\"],\"version\":\"1.0\"}"
  Angles Estimation : MATLAB Function  TreatAsAtomicUnit=on
  Bus Selector1 : BusSelector  OutputSignals=x,y,z,vx,vy,vz,ax,ay,az,ref_lat,ref_lon,ref_alt
  Bus Selector10 : BusSelector  OutputSignals=ifr_nav_active
  Bus Selector2 : BusSelector  OutputSignals=xyz
  Bus Selector3 : BusSelector  OutputSignals=north_east,track,speeds,acc_k,attitude,rates,actuator,ref_lla,asl
  Bus Selector4 : BusSelector  OutputSignals=indicated_airspeed_m_s
  Bus Selector5 : BusSelector  OutputSignals=q
  Bus Selector6 : BusSelector  OutputSignals=nav.xi_max,nav.eta_max,nav.zeta_max
  Bus Selector7 : BusSelector  OutputSignals=xi_max,eta_max,zeta_max
  Bus Selector8 : BusSelector  OutputSignals=rc_mode
  Bus Selector9 : BusSelector  OutputSignals=trk_der_switch
  Data Type Conversion : DataTypeConversion  OutDataTypeStr=single  SaturateOnIntegerOverflow=off  RndMeth=Floor
  Data Type Conversion1 : DataTypeConversion  OutDataTypeStr=single  SaturateOnIntegerOverflow=off  RndMeth=Floor
  Demux11 : Demux  Outputs=2
  Demux12 : Demux  Outputs=3
  Gain : Gain  Gain=[1e-7,1e-7,1e-3]
  MATLAB Function : MATLAB Function  TreatAsAtomicUnit=on
  MATLAB Function2 : MATLAB Function  TreatAsAtomicUnit=on
  Minus{,1..11} (12 alike) : Sum  Inputs=+-
  Mux{,1..2,4..5} (5 alike) : Mux  Inputs=3
  Mux3 : Mux  Inputs=2
  Mux6 : Mux  Inputs=5
  Scope{,1..11} (12 alike) : Scope  NumInputPorts=3
      Scope settings: ActiveDisplayYMinimum=-2.6480022855103016  ActiveDisplayYMaximum=0.52406292036175728  DataLoggingVariableName=ScopeData14
      Scope1 settings: ActiveDisplayYMinimum=-24.382436275482178  ActiveDisplayYMaximum=24.385049343109131  DataLoggingVariableName=ScopeData15
      Scope10 settings: ActiveDisplayYMinimum=1  ActiveDisplayYMaximum=3  DataLoggingVariableName=ScopeData27
      Scope11 settings: ActiveDisplayYMinimum=-1.4540479779243469  ActiveDisplayYMaximum=1.7983081927498716  DataLoggingVariableName=ScopeData28
      Scope2 settings: ActiveDisplayYMinimum=-2.8663190840743478  ActiveDisplayYMaximum=26.245877308305353  DataLoggingVariableName=ScopeData17
      Scope3 settings: ActiveDisplayYMinimum=-2.4921854510903358  ActiveDisplayYMaximum=0.56816831976175308  DataLoggingVariableName=ScopeData18
      Scope4 settings: ActiveDisplayYMinimum=-2713.6547136306763  ActiveDisplayYMaximum=421.09798908233637  DataLoggingVariableName=ScopeData19
      Scope5 settings: ActiveDisplayYMinimum=-0.12499999999999997  ActiveDisplayYMaximum=1.125  DataLoggingVariableName=ScopeData20
      Scope6 settings: ActiveDisplayYMinimum=-399.43122087977827  ActiveDisplayYMaximum=44.557806765660636  DataLoggingVariableName=ScopeData22
      Scope7 settings: ActiveDisplayYMinimum=354616.43457077962  ActiveDisplayYMaximum=354997.88472456852  DataLoggingVariableName=ScopeData23
      Scope8 settings: ActiveDisplayYMinimum=-0.53752770274877548  ActiveDisplayYMaximum=1.1725589856505394  DataLoggingVariableName=ScopeData25
      Scope9 settings: ActiveDisplayYMinimum=-1.1700206249952316  ActiveDisplayYMaximum=1.1303310841321945  DataLoggingVariableName=ScopeData26
  Scope12 : Scope  NumInputPorts=12
      settings: ActiveDisplayYMinimum=-0.30250503619950209  ActiveDisplayYMaximum=1.2360685245310084  DataLoggingVariableName=ScopeData35
  Subsystem : Subsystem
      settings: PortSchema="{\"entries\":[{\"content\":{\"sides\":[{\"content\":{\"connectorIds\":[\"In1\",\"In2\",\"In3\"]},\"type\":\"ConnectorPlacement.EquallySpacedRectSide\",\"uuid\":\"d3f70b0d-5808-41a1-901a-3e2b7a37eb93\"},{\"content\":{\"connectorIds\":[\"Out1\"],\"side\":\"RIGHT\"},\"type\":\"ConnectorPlacement.EquallySpacedRectSide\",\"uuid\":\"dc4ca20c-eb1b-4454-88d2-269a48f937e4\"},{\"content\":{\"connectorIds\":[\"In4\"],\"side\":\"TOP\"},\"type\":\"ConnectorPlacement.EquallySpacedRectSide\",\"uuid\":\"1dace743-43be-4004-9081-e38a97e7a582\"}]},\"type\":\"ConnectorPlacement.EquallySpacedConnector\",\"uuid\":\"5771c896-d5ee-401f-a70a-0ba475a64d58\"}],\"packageUris\":[\"http://schema.mathworks.com/mf0/Connector/R2020b\"],\"version\":\"1.0\"}"
  Subsystem1 : Subsystem
      settings: PortSchema="{\"entries\":[{\"content\":{\"sides\":[{\"content\":{\"connectorIds\":[\"In1\",\"In2\"]},\"type\":\"ConnectorPlacement.EquallySpacedRectSide\",\"uuid\":\"5ad240f1-9900-4302-9829-f7f76c92f7f3\"},{\"content\":{\"connectorIds\":[\"Out1\"],\"side\":\"RIGHT\"},\"type\":\"ConnectorPlacement.EquallySpacedRectSide\",\"uuid\":\"2e078b74-c070-4ff4-9462-14d77c7ea852\"},{\"content\":{\"connectorIds\":[\"In3\"],\"side\":\"TOP\"},\"type\":\"ConnectorPlacement.EquallySpacedRectSide\",\"uuid\":\"8333c2e0-27a1-46ea-af37-c72f43f5eec5\"},{\"content\":{\"side\":\"BOTTOM\"},\"type\":\"ConnectorPlacement.EquallySpacedRectSide\",\"uuid\":\"a97c1683-6bc4-4c28-a612-acefec17359f\"}]},\"type\":\"ConnectorPlacement.EquallySpacedConnector\",\"uuid\":\"336c4d27-e0be-411f-89e0-bb484511dd68\"}],\"packageUris\":[\"http://schema.mathworks.com/mf0/Connector/R2020b\"],\"version\":\"1.0\"}"
  Subsystem2 : Subsystem
      settings: PortSchema="{\"entries\":[{\"content\":{\"sides\":[{\"content\":{\"connectorIds\":[\"In1\"]},\"type\":\"ConnectorPlacement.EquallySpacedRectSide\",\"uuid\":\"c249bde2-4580-435b-8669-29d5f206d176\"},{\"content\":{\"connectorIds\":[\"Out1\"],\"side\":\"RIGHT\"},\"type\":\"ConnectorPlacement.EquallySpacedRectSide\",\"uuid\":\"60962190-2f64-42e9-bf1a-6d4a20eea6b3\"},{\"content\":{\"side\":\"TOP\"},\"type\":\"ConnectorPlacement.EquallySpacedRectSide\",\"uuid\":\"d4f64458-133b-4324-95a6-14c38555dd9a\"},{\"content\":{\"connectorIds\":[\"In2\"],\"side\":\"BOTTOM\"},\"type\":\"ConnectorPlacement.EquallySpacedRectSide\",\"uuid\":\"5ed7f531-edd6-4543-875a-2dd5af02d360\"}]},\"type\":\"ConnectorPlacement.EquallySpacedConnector\",\"uuid\":\"8eaaea99-2870-4f7f-ab6c-9598fb8c4fc7\"}],\"packageUris\":[\"http://schema.mathworks.com/mf0/Connector/R2020b\"],\"version\":\"1.0\"}"
  Subsystem3 : Subsystem
  Switch{,1..12} (13 alike) : Switch  Criteria=u2 > Threshold  SaturateOnIntegerOverflow=off  InputSameDT=off
  acc transformation : MATLAB Function  TreatAsAtomicUnit=on
  acc transformation4 : MATLAB Function  TreatAsAtomicUnit=on
  ref_LLA : Outport
  <north_east> : Outport  Port=2
  ASL : Outport  Port=3
  rc_mode : Outport  Port=4  OutDataTypeStr=uint8  PortDimensions=1
  <track> : Outport  Port=5
  <speeds> : Outport  Port=6
  <acc_k> : Outport  Port=7
  <attitude> : Outport  Port=8
  <rates> : Outport  Port=9
  <actuator> : Outport  Port=10
  act_limits : Outport  Port=11
  trk_deriv : Outport  Port=12  PortDimensions=2
  RC_trim : Outport  Port=13  PortDimensions=4
  acc_moni : Outport  Port=14  OutDataTypeStr=Bus: accel_monitor_bus
  wires:
  Bus Selector9/1 -> Subsystem2/2(trk_deriv_sw), Subsystem/4(trk_deriv_sw)  "<trk_der_switch>"
  RC_trim_in/1 -> Subsystem3/1(RC_trim)
  track_deriv/1 -> Subsystem2/1(track_deriv)
  Subsystem1/1(acc_moni) -> acc_moni/1
  acc transformation4/1(acc_g) -> Subsystem1/2(acc_g_filt)  "Am"
  MATLAB Function2/2(acc_b) -> acc transformation4/1(acc_b)
  Subsystem/1(d_trk_moni) -> Minus10/2, Scope11/2, Switch12/3
  Subsystem2/1(trk_deriv) -> Scope11/1, Minus10/1, Switch12/1
  Switch12/1 -> Scope11/3, trk_deriv/1
  Subsystem3/1(rc_controls) -> Minus9/1, Scope5/1, Switch11/1
  Switch11/1 -> Scope5/3, RC_trim/1
  Actuator_Model/3(rc_trim) -> Minus9/2, Scope5/2, Switch11/3
  Data Type Conversion1/1 -> Mux2/2
  Data Type Conversion/1 -> Mux2/1
  Mux2/1 -> Scope7/2, Minus7/2, Switch7/3
  Bus Selector8/1 -> Minus11/1, Scope10/1, Switch10/1  "<rc_mode>"
  acc_filt/1 -> MATLAB Function2/3(acc_filt)
  accel/1 -> MATLAB Function2/2(acc_raw)
  MATLAB Function2/1(aero_est) -> Demux11/1
  Mux6/1 -> Minus4/2, Scope/2, Switch4/3
  Demux12/2 -> Mux6/2
  Demux12/3 -> Mux6/4
  Demux11/1 -> Mux6/1
  Demux11/2 -> Mux6/3
  Demux12/1 -> Mux6/5
  Switch10/1 -> Scope10/3, rc_mode/1
  RC_mde/1 -> Bus Selector8/1
  Actuator_Model/2(rc_mode) -> Scope10/2, Minus11/2, Switch10/3
  Mux5/1 -> Switch9/1
  Bus Selector7/3 -> Mux5/3  "<zeta_max>"
  Bus Selector7/2 -> Mux5/2  "<eta_max>"
  Bus Selector7/1 -> Mux5/1  "<xi_max>"
  Bus Selector6/3 -> Mux4/3  "<zeta_max>"
  Bus Selector6/2 -> Mux4/2  "<eta_max>"
  Bus Selector6/1 -> Mux4/1  "<xi_max>"
  Mux4/1 -> Switch9/3
  para_gnc/1 -> MATLAB Function2/1(param), Bus Selector10/1, Bus Selector9/1, Bus Selector6/1
  Bus Selector10/1 -> Switch8/2, Switch10/2, Switch9/2, Switch12/2, Switch11/2, Switch7/2, Switch6/2, Switch5/2, Switch4/2, Switch3/2, Switch2/2, Switch1/2, Switch/2  "<ifr_nav_active>"
  Switch9/1 -> act_limits/1, Actuator_Model/3(act_lims)
  act_lims/1 -> Bus Selector7/1
  main_axes/1 -> Actuator_Model/2(main_axes)
  rc_channel/1 -> Actuator_Model/1(rc_channel)
  Bus Selector1/3 -> Minus8/2, Scope6/2, Switch8/3  "<z>"
  Bus Selector1/12 -> Mux2/3  "<ref_alt>"
  Bus Selector1/11 -> Data Type Conversion1/1  "<ref_lon>"
  Bus Selector1/10 -> Data Type Conversion/1  "<ref_lat>"
  Actuator_Model/1(act_m) -> Minus6/2, Scope8/2, Switch6/3
  Switch7/1 -> Scope7/3, ref_LLA/1
  Switch6/1 -> Scope8/3, <actuator>/1
  Switch8/1 -> Scope6/3, ASL/1
  Switch5/1 -> Scope9/3, <rates>/1
  Switch4/1 -> Scope/3, <attitude>/1
  Switch3/1 -> Scope1/3, <acc_k>/1
  Switch2/1 -> Scope2/3, <speeds>/1
  Switch1/1 -> Scope3/3, <track>/1
  Switch/1 -> Scope4/3, <north_east>/1
  Bus Selector3/9 -> Minus8/1, Scope6/1, Switch8/1  "<asl>"
  Bus Selector3/8 -> Minus7/1, Scope7/1, Switch7/1  "<ref_lla>"
  Mux3/1 -> Minus/2, Scope4/2, Switch/3
  Angles Estimation/1(speeds) -> Minus2/2, Scope2/2, Switch2/3, Subsystem/1(speeds)
  MATLAB Function/1(eul_rad) -> acc transformation4/2(euler), Demux12/1, Angles Estimation/1(euler)
  Mux1/1 -> acc transformation/2(acc_g), Subsystem1/1(acc_g_vlp)
  Bus Selector1/9 -> Mux1/3  "<az>"
  Bus Selector1/8 -> Mux1/2  "<ay>"
  Bus Selector1/7 -> Mux1/1  "<ax>"
  Bus Selector1/1 -> Mux3/1  "<x>"
  Mux/1 -> Angles Estimation/2(vel)
  Bus Selector1/6 -> Mux/3  "<vz>"
  vehicle_pos/1 -> Bus Selector1/1
  Bus Selector1/4 -> Mux/1  "<vx>"
  airspeed/1 -> Bus Selector4/1
  Bus Selector1/5 -> Mux/2  "<vy>"
  Bus Selector4/1 -> Angles Estimation/3(Va)  "<indicated_airspeed_m_s>"
  vehicle_ang_vel/1 -> Bus Selector2/1
  Bus Selector1/2 -> Mux3/2  "<y>"
  Bus Selector5/1 -> MATLAB Function/1(quat)  "<q>"
  vehicle_att/1 -> Bus Selector5/1
  Angles Estimation/2(track) -> Minus1/2, Switch1/3, Scope3/2, acc transformation/1(gachi_m), Subsystem/2(track)
  Bus Selector2/1 -> Scope9/2, Minus5/2, Switch5/3  "<xyz>"
  vehicle_state/1 -> Bus Selector3/1
  Bus Selector3/3 -> Minus2/1, Scope2/1, Switch2/1  "<speeds>"
  Bus Selector3/6 -> Minus5/1, Scope9/1, Switch5/1  "<rates>"
  Bus Selector3/2 -> Minus1/1, Scope3/1, Switch1/1  "<track>"
  Bus Selector3/1 -> Minus/1, Scope4/1, Switch/1  "<north_east>"
  Bus Selector3/7 -> Minus6/1, Scope8/1, Switch6/1  "<actuator>"
  Bus Selector3/4 -> Minus3/1, Scope1/1, Switch3/1  "<acc_k>"
  Bus Selector3/5 -> Minus4/1, Scope/1, Switch4/1  "<attitude>"
  acc transformation/1(acc_k) -> Subsystem/3(acc_k), Minus3/2, Scope1/2, Switch3/3, Subsystem1/3(acc_k)
  Minus/1 -> Scope12/1
  Minus1/1 -> Scope12/2
  Minus2/1 -> Scope12/3
  Minus3/1 -> Scope12/4
  Minus4/1 -> Scope12/5
  Minus5/1 -> Scope12/6
  Minus6/1 -> Scope12/7
  Minus7/1 -> Gain/1
  Minus8/1 -> Scope12/9
  Minus9/1 -> Scope12/10
  Minus10/1 -> Scope12/11
  Minus11/1 -> Scope12/12
  Gain/1 -> Scope12/8

== system gnc/bus_generator ==
  axis_modes : Inport
  RC_trim : Inport  Port=2
  rc_mode : Inport  Port=3
  Bus Creator : BusCreator  Inputs=10  OutDataTypeStr=Bus: rc_gnc_output_bus
      settings: InheritFromInputs=off
  Demux : Demux
  Demux1 : Demux
  is_valid : Constant  Value=0  OutDataTypeStr=boolean
  RC_gnc_output : Outport  OutDataTypeStr=Bus: rc_gnc_output_bus
  wires:
  is_valid/1 -> Bus Creator/1
  Bus Creator/1 -> RC_gnc_output/1
  RC_trim/1 -> Demux/1
  axis_modes/1 -> Demux1/1
  Demux/1 -> Bus Creator/2
  Demux/2 -> Bus Creator/3
  Demux/3 -> Bus Creator/4
  Demux/4 -> Bus Creator/5
  Demux1/2 -> Bus Creator/7
  Demux1/3 -> Bus Creator/8
  Demux1/4 -> Bus Creator/9
  Demux1/1 -> Bus Creator/6
  rc_mode/1 -> Bus Creator/10

== system gnc/INDI/Attitude ==
  note: alpha
      | theta
      | beta
      | psi
      | mu
  param : Inport  OutDataTypeStr=Bus: gnc_parameterBus
  att_direct : Inport  Port=2
  roll_lim : Inport  Port=3  OutDataTypeStr=single  PortDimensions=1
  d/dt_gachiv_m : Inport  Port=4  OutDataTypeStr=single  PortDimensions=3
  att_ctrl : Inport  Port=5
  gachi_m : Inport  Port=6
  att_m : Inport  Port=7
  axis_modes : Inport  Port=8
  MATLAB Function : MATLAB Function  TreatAsAtomicUnit=on
  Nonlinear_inversion : Subsystem
  Pseudo-control : Subsystem
  pqr_c : Outport
  att_moni : Outport  Port=2  OutDataTypeStr=single  PortDimensions=20
  wires:
  att_m/1 -> Pseudo-control/3(att_m), Nonlinear_inversion/3(att_m)
  param/1 -> Nonlinear_inversion/2(param), Pseudo-control/4(param)
  d/dt_gachiv_m/1 -> Nonlinear_inversion/5(d/dt_gachiv_m)
  gachi_m/1 -> Nonlinear_inversion/6(path_m)
  MATLAB Function/1(att_c) -> Pseudo-control/1(att_c)
  Nonlinear_inversion/1(rates_ltd) -> pqr_c/1
  Pseudo-control/2(d/dt_att_c) -> Nonlinear_inversion/1(d/dt_att_c)
  Pseudo-control/1(att_moni) -> att_moni/1
  roll_lim/1 -> Pseudo-control/2(roll_lim)
  axis_modes/1 -> Nonlinear_inversion/4(modes), MATLAB Function/3(modes)
  att_ctrl/1 -> MATLAB Function/2(guidance)
  att_direct/1 -> MATLAB Function/1(direct)
